simulink subsystem "FOC_Sub_CoreAlgoithm"  (R2020b)
settings: Solver=VariableStepAuto  StartTime=0.0  StopTime=10.0  RelTol=1e-3
PreLoadFcn:
  | FOC_Config;
values from neighbouring files (symbols this model uses):
  CurrentLoopMax = 1.2    [FOC_Config.m]
  fluxF = Lam_realvalue/fluxB    [FOC_Config.m]
  Id_Ki = CurrentLoopBandwidth*Rs    [FOC_Config.m]
  Id_Kp = CurrentLoopBandwidth*Ld    [FOC_Config.m]
  Iq_Ki = CurrentLoopBandwidth*Rs    [FOC_Config.m]
  Iq_Kp = CurrentLoopBandwidth*Lq    [FOC_Config.m]
  Ld = Ld_realvalue/Lb    [FOC_Config.m]
  Lq = Lq_realvalue/Lb    [FOC_Config.m]
  Omega0 = 0.4    [PLLObserver.sldd]
  PLL_KI = PLL_Bandwidth*PLL_Bandwidth    (= 0.16)    [FOC_Config.m]
  PLL_KP = 2*PLL_Bandwidth    (= 0.8)    [FOC_Config.m]
  PLL_OUTMax_W = 1.2    [FOC_Config.m]
  Rs = Rs_realvalue/Rb    [FOC_Config.m]
  tb = 1/Wb    (= 0.000636619772368)    [FOC_Config.m]
  Ts = 1/SwitchFrequency    (= 6.25e-05)    [FOC_Config.m]
  Wb = 2*pi*fn    (= 1570.79632679)    [FOC_Config.m]
undefined symbols (not defined in the file or in its folder): DiscIntNeverNeededParam, motor
libraries: mcbcontrolslib x2
settings Model: Creator=k  LastModifiedBy=wangdi

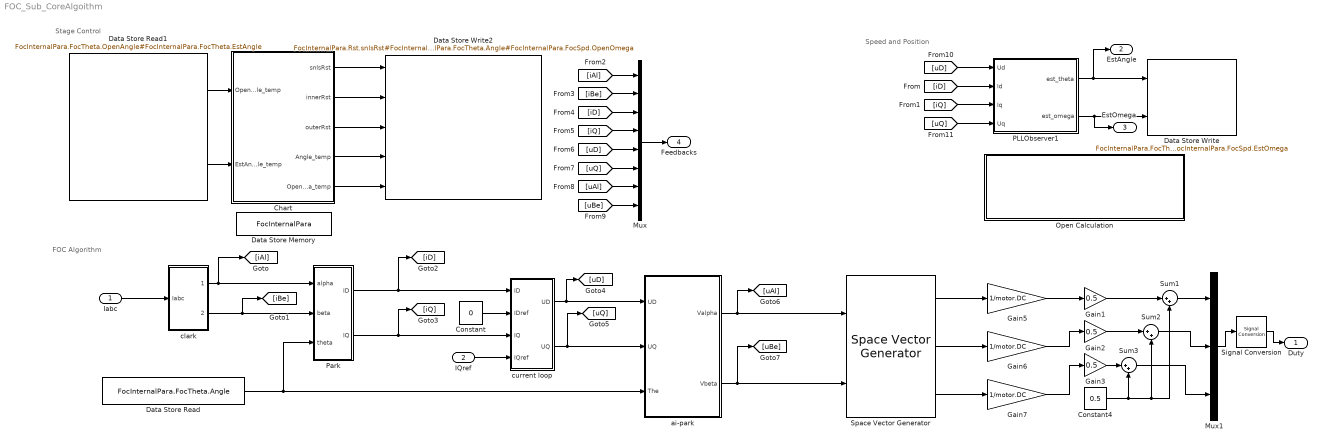
== system FOC_Sub_CoreAlgoithm ==
  note: FOC Algorithm
  note: Stage Control
  note: Speed and Position
  Iabc : Inport
  IQref : Inport  Port=2
  Chart : Stateflow chart  TreatAsAtomicUnit=on
  Constant : Constant  Value=0  OutDataTypeStr=single
  Constant4 : Constant  Value=0.5  OutDataTypeStr=single
  Data Store Memory : DataStoreMemory  DataStoreName=FocInternalPara  ReadBeforeWriteMsg=warning  WriteAfterWriteMsg=warning  WriteAfterReadMsg=warning  ShowAdditionalParam=off  OutDataTypeStr=Bus: strcutFocInternalPara
  Data Store Read : DataStoreRead  DataStoreName=FocInternalPara  DataStoreElements=FocInternalPara.FocTheta.Angle
  Data Store Read1 : DataStoreRead  DataStoreName=FocInternalPara  DataStoreElements=FocInternalPara.FocTheta.OpenAngle#FocInternalPara.FocTheta.EstAngle
  Data Store Write : DataStoreWrite  DataStoreName=FocInternalPara  DataStoreElements=FocInternalPara.FocTheta.EstAngle#FocInternalPara.FocSpd.EstOmega
  Data Store Write2 : DataStoreWrite  DataStoreName=FocInternalPara  DataStoreElements=FocInternalPara.Rst.snlsRst#FocInternalPara.Rst.innerCtrRst#FocInternalPara.Rst.outerRst#FocInternalPara.FocTheta.Angle#FocInternalPara.FocSpd.OpenOmega
  Gain1 : Gain  Gain=0.5  OutDataTypeStr=single
  Gain2 : Gain  Gain=0.5  OutDataTypeStr=single
  Gain3 : Gain  Gain=0.5  OutDataTypeStr=single
  Gain5 : Gain  Gain=1/motor.DC
  Gain6 : Gain  Gain=1/motor.DC
  Gain7 : Gain  Gain=1/motor.DC
  Mux : Mux  Inputs=8
  Mux1 : Mux  Inputs=3
  Open Calculation : Subsystem
  PLLObserver1 : Subsystem  TreatAsAtomicUnit=on
      settings: RTWFcnNameOpts=Use subsystem name  RTWFileNameOpts=Use subsystem name
  Park : Subsystem
  Signal Conversion : SignalConversion  OverrideOpt=off
  Space Vector Generator : mcbcontrolslib/Space Vector Generator
      settings: SourceProductBaseCode=MT
  Sum1 : Sum  Inputs=|++
  Sum2 : Sum  Inputs=|++
  Sum3 : Sum  Inputs=|++
  ai-park : Subsystem
  clark : Subsystem
  current loop : Subsystem
  Duty : Outport  PortDimensions=3
  EstAngle : Outport  Port=2
  EstOmega : Outport  Port=3
  Feedbacks : Outport  Port=4
  wires:
  Constant/1 -> current loop/2(IDref)
  Park/1(ID) -> [iD], current loop/1(ID)
  Iabc/1 -> clark/1(Iabc)
  Mux/1 -> Feedbacks/1
  [iAl] -> Mux/1
  [iBe] -> Mux/2
  [iD] -> Mux/3
  [iQ] -> Mux/4
  [uD] -> Mux/5
  [uQ] -> Mux/6
  [uAl] -> Mux/7
  [uBe] -> Mux/8
  [uQ] -> PLLObserver1/4(Uq)
  [uD] -> PLLObserver1/1(Ud)
  [iQ] -> PLLObserver1/3(Iq)
  [iD] -> PLLObserver1/2(Id)
  Chart/5(OpenOmega_temp) -> Data Store Write2/5
  Chart/4(Angle_temp) -> Data Store Write2/4
  Data Store Read1/2 -> Chart/2(EstAngle_temp)
  Data Store Read1/1 -> Chart/1(OpenAngle_temp)
  Chart/1(snlsRst) -> Data Store Write2/1
  Chart/2(innerRst) -> Data Store Write2/2
  Chart/3(outerRst) -> Data Store Write2/3
  Data Store Read/1 -> ai-park/3(The), Park/3(theta)
  current loop/2(UQ) -> ai-park/2(UQ), [uQ]
  current loop/1(UD) -> ai-park/1(UD), [uD]
  Park/2(IQ) -> [iQ], current loop/3(IQ)
  ai-park/2(Vbeta) -> [uBe], Space Vector Generator/2
  ai-park/1(Valpha) -> [uAl], Space Vector Generator/1
  Gain6/1 -> Gain2/1
  Gain3/1 -> Sum3/1
  Gain2/1 -> Sum2/1
  Space Vector Generator/3 -> Gain7/1
  Gain1/1 -> Sum1/1
  Gain5/1 -> Gain1/1
  Space Vector Generator/2 -> Gain6/1
  Space Vector Generator/1 -> Gain5/1
  Constant4/1 -> Sum1/2, Sum2/2, Sum3/2
  Gain7/1 -> Gain3/1
  clark/2(Ibeta) -> Park/2(beta), [iBe]
  clark/1(Ialpha) -> [iAl], Park/1(alpha)
  Sum2/1 -> Mux1/2
  Sum3/1 -> Mux1/3
  Sum1/1 -> Mux1/1
  Mux1/1 -> Signal Conversion/1
  Signal Conversion/1 -> Duty/1
  IQref/1 -> current loop/4(IQref)
  PLLObserver1/2(est_omega) -> Data Store Write/2, EstOmega/1
  PLLObserver1/1(est_theta) -> Data Store Write/1, EstAngle/1

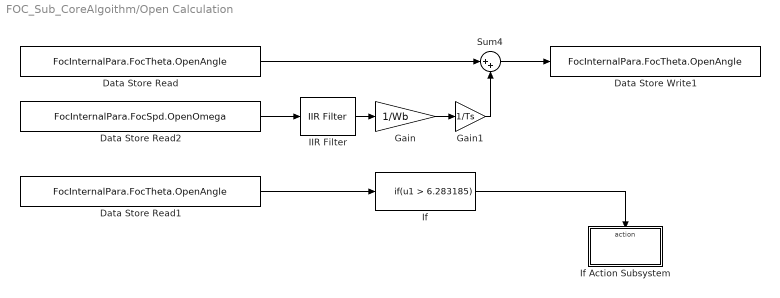
== system FOC_Sub_CoreAlgoithm/Open Calculation ==
  Data Store Read : DataStoreRead  DataStoreName=FocInternalPara  DataStoreElements=FocInternalPara.FocTheta.OpenAngle
  Data Store Read1 : DataStoreRead  DataStoreName=FocInternalPara  DataStoreElements=FocInternalPara.FocTheta.OpenAngle
  Data Store Read2 : DataStoreRead  DataStoreName=FocInternalPara  DataStoreElements=FocInternalPara.FocSpd.OpenOmega
  Data Store Write1 : DataStoreWrite  DataStoreName=FocInternalPara  DataStoreElements=FocInternalPara.FocTheta.OpenAngle
  Gain : Gain  Gain=1/Wb
  Gain1 : Gain  Gain=1/Ts
  IIR Filter : mcbcontrolslib/IIR Filter  Filter_constant=0.002
      settings: SourceProductBaseCode=MT
  If : If  IfExpression=u1 > 6.283185  ShowElse=off
  If Action Subsystem : Subsystem  TreatAsAtomicUnit=on
  Sum4 : Sum  Inputs=|++  OutDataTypeStr=single
  wires:
  Gain1/1 -> Sum4/2
  Gain/1 -> Gain1/1
  IIR Filter/1 -> Gain/1
  Data Store Read2/1 -> IIR Filter/1
  Sum4/1 -> Data Store Write1/1
  Data Store Read/1 -> Sum4/1
  Data Store Read1/1 -> If/1
  If/1 -> If Action Subsystem/Action

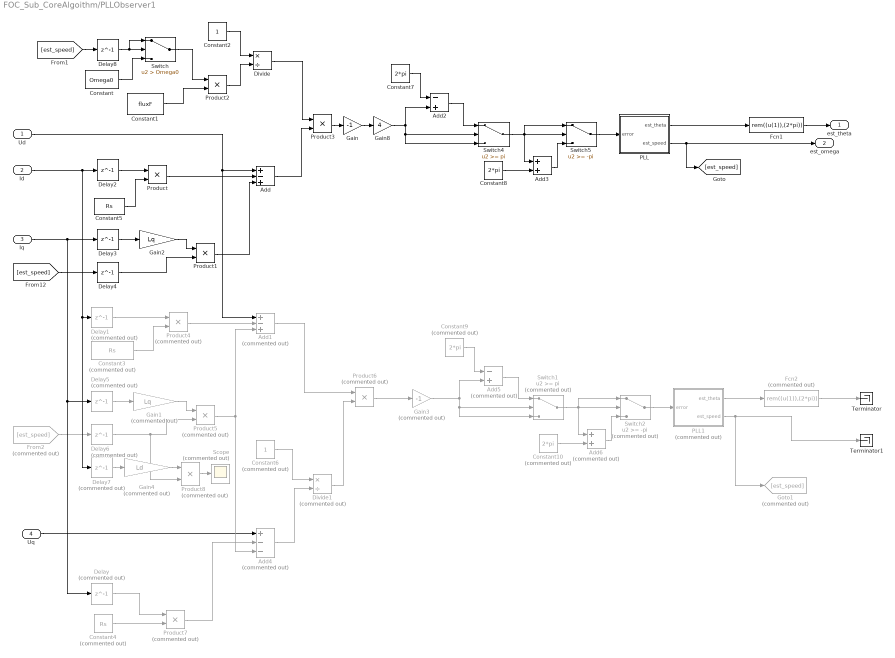
== system FOC_Sub_CoreAlgoithm/PLLObserver1 ==
  Ud : Inport
  Id : Inport  Port=2
  Iq : Inport  Port=3
  Uq : Inport  Port=4
  Add : Sum  Inputs=+-+
  Add1 : Sum  Commented=on  Inputs=+-+
  Add2 : Sum  Inputs=-+
  Add3 : Sum
  Add4 : Sum  Commented=on  Inputs=+--
  Add5 : Sum  Commented=on  Inputs=-+
  Add6 : Sum  Commented=on
  Constant : Constant  Value=Omega0  OutDataTypeStr=single
  Constant1 : Constant  Value=fluxF  OutDataTypeStr=single
  Constant10 : Constant  Commented=on  Value=2*pi
  Constant2 : Constant  OutDataTypeStr=single
  Constant3 : Constant  Commented=on  Value=Rs  OutDataTypeStr=single
  Constant4 : Constant  Commented=on  Value=Rs  OutDataTypeStr=single
  Constant5 : Constant  Value=Rs  OutDataTypeStr=single
  Constant6 : Constant  Commented=on  OutDataTypeStr=single
  Constant7 : Constant  Value=2*pi  OutDataTypeStr=single
  Constant8 : Constant  Value=2*pi  OutDataTypeStr=single
  Constant9 : Constant  Commented=on  Value=2*pi  OutDataTypeStr=single
  Delay{,1,5..7} (5 alike) : Delay  Commented=on  DelayLength=1
  Delay{2..4,8} (4 alike) : Delay  DelayLength=1
  Divide : Product  Inputs=*/
  Divide1 : Product  Commented=on  Inputs=*/
  Fcn1 : Fcn  Expr=rem((u(1)),(2*pi))
  Fcn2 : Fcn  Commented=on  Expr=rem((u(1)),(2*pi))
  From2 : From  Commented=on  GotoTag=est_speed
  Gain : Gain  Gain=-1
  Gain1 : Gain  Commented=on  Gain=Lq
  Gain2 : Gain  Gain=Lq
  Gain3 : Gain  Commented=on  Gain=-1
  Gain4 : Gain  Commented=on  Gain=Ld
  Gain8 : Gain  Gain=4
  Goto1 : Goto  Commented=on  GotoTag=est_speed
  PLL : Subsystem  TreatAsAtomicUnit=on
  PLL1 : Subsystem  Commented=on
  Product{,1..3} (4 alike) : Product
  Product{4..8} (5 alike) : Product  Commented=on
  Scope : Scope  Commented=on
  Switch : Switch  Criteria=u2 > Threshold  Threshold=Omega0
  Switch1 : Switch  Commented=on  Threshold=pi
  Switch2 : Switch  Commented=on  Threshold=-pi
  Switch4 : Switch  Threshold=pi
  Switch5 : Switch  Threshold=-pi
  Terminator : Terminator
  Terminator1 : Terminator
  est_theta : Outport
  est_omega : Outport  Port=2
  wires:
  [est_speed] -> Delay8/1
  PLL/1(est_theta) -> Fcn1/1
  Gain8/1 -> Add2/2, Switch4/2, Switch4/3
  Add/1 -> Product3/2
  Product1/1 -> Add/3
  Product/1 -> Add/2
  Product8/1 -> Scope/1
  Gain4/1 -> Product8/1
  From2/1 -> Delay6/1
  Delay7/1 -> Gain4/1
  Fcn1/1 -> est_theta/1
  PLL1/2(est_speed) -> Goto1/1, Terminator1/1
  Fcn2/1 -> Terminator/1
  PLL1/1(est_theta) -> Fcn2/1
  Add6/1 -> Switch2/3
  Gain3/1 -> Add5/2, Switch1/2, Switch1/3
  Add5/1 -> Switch1/1
  Switch2/1 -> PLL1/1(error)
  Constant10/1 -> Add6/2
  Constant9/1 -> Add5/1
  Switch1/1 -> Switch2/2, Add6/1, Switch2/1
  Product6/1 -> Gain3/1
  Divide1/1 -> Product6/2
  Add4/1 -> Divide1/2
  Constant6/1 -> Divide1/1
  Product7/1 -> Add4/2
  Constant4/1 -> Product7/2
  Delay/1 -> Product7/1
  Uq/1 -> Add4/1
  Add1/1 -> Product6/1
  Product5/1 -> Add1/3, Add4/3
  Iq/1 -> Delay3/1, Delay5/1, Delay/1
  Delay5/1 -> Gain1/1
  Gain1/1 -> Product5/1
  Delay6/1 -> Product5/2, Product8/2
  Ud/1 -> Add/1, Add1/1
  Delay1/1 -> Product4/1
  Product4/1 -> Add1/2
  Constant3/1 -> Product4/2
  Gain/1 -> Gain8/1
  Product3/1 -> Gain/1
  Switch5/1 -> PLL/1(error)
  Add2/1 -> Switch4/1
  Constant7/1 -> Add2/1
  Constant8/1 -> Add3/2
  Add3/1 -> Switch5/3
  PLL/2(est_speed) -> [est_speed], est_omega/1
  Switch4/1 -> Switch5/2, Add3/1, Switch5/1
  Divide/1 -> Product3/1
  Product2/1 -> Divide/2
  Constant2/1 -> Divide/1
  Constant1/1 -> Product2/2
  Switch/1 -> Product2/1
  Constant/1 -> Switch/3
  Delay8/1 -> Switch/2, Switch/1
  Id/1 -> Delay2/1, Delay1/1, Delay7/1
  Delay2/1 -> Product/1
  Delay3/1 -> Gain2/1
  Gain2/1 -> Product1/1
  Delay4/1 -> Product1/2
  [est_speed] -> Delay4/1
  Constant5/1 -> Product/2

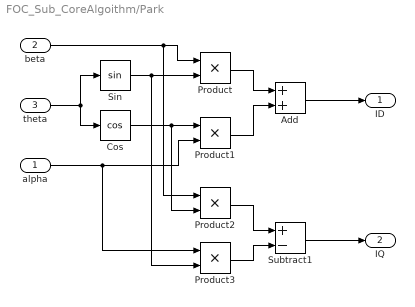
== system FOC_Sub_CoreAlgoithm/Park ==
  alpha : Inport
  beta : Inport  Port=2
  theta : Inport  Port=3
  Add : Sum  OutDataTypeStr=single
  Cos : Trigonometry  Operator=cos
  Product{,1..3} (4 alike) : Product
  Sin : Trigonometry
  Subtract1 : Sum  Inputs=+-  OutDataTypeStr=single
  ID : Outport
  IQ : Outport  Port=2
  wires:
  Product2/1 -> Subtract1/1
  beta/1 -> Product2/1, Product/1
  theta/1 -> Cos/1, Sin/1
  Sin/1 -> Product3/2, Product/2
  alpha/1 -> Product3/1, Product1/2
  Cos/1 -> Product1/1, Product2/2
  Subtract1/1 -> IQ/1
  Product1/1 -> Add/2
  Product3/1 -> Subtract1/2
  Product/1 -> Add/1
  Add/1 -> ID/1

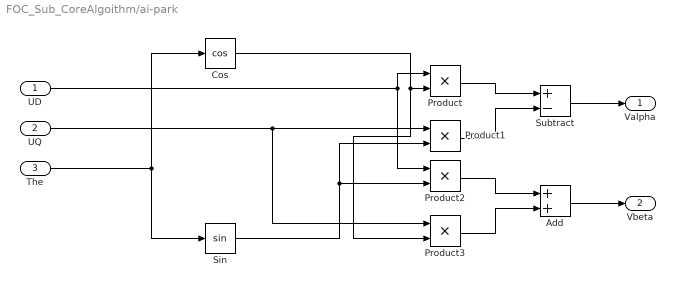
== system FOC_Sub_CoreAlgoithm/ai-park ==
  UD : Inport
  UQ : Inport  Port=2
  The : Inport  Port=3
  Add : Sum
  Cos : Trigonometry  Operator=cos
  Product{,1..3} (4 alike) : Product
  Sin : Trigonometry
  Subtract : Sum  Inputs=+-
  Valpha : Outport
  Vbeta : Outport  Port=2
  wires:
  Add/1 -> Vbeta/1
  Subtract/1 -> Valpha/1
  UD/1 -> Product2/1, Product/1
  The/1 -> Cos/1, Sin/1
  Product2/1 -> Add/1
  Product/1 -> Subtract/1
  Sin/1 -> Product1/2, Product2/2
  Cos/1 -> Product/2, Product3/2
  Product3/1 -> Add/2
  Product1/1 -> Subtract/2
  UQ/1 -> Product1/1, Product3/1

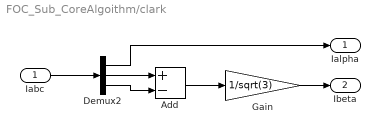
== system FOC_Sub_CoreAlgoithm/clark ==
  Iabc : Inport  OutDataTypeStr=single
  Add : Sum  Inputs=+-
  Demux2 : Demux  Outputs=3
  Gain : Gain  Gain=1/sqrt(3)
  Ialpha : Outport
  Ibeta : Outport  Port=2
  wires:
  Demux2/3 -> Add/2
  Demux2/1 -> Ialpha/1
  Demux2/2 -> Add/1
  Iabc/1 -> Demux2/1
  Add/1 -> Gain/1
  Gain/1 -> Ibeta/1

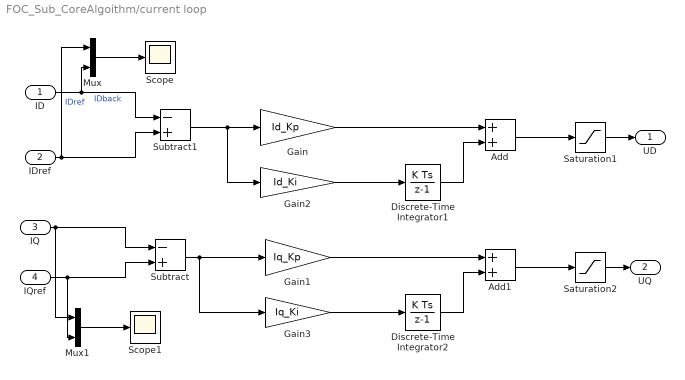
== system FOC_Sub_CoreAlgoithm/current loop ==
  ID : Inport  OutDataTypeStr=single
  IDref : Inport  Port=2  OutDataTypeStr=single
  IQ : Inport  Port=3  OutDataTypeStr=single
  IQref : Inport  Port=4  OutDataTypeStr=single
  Add : Sum
  Add1 : Sum
  Discrete-Time Integrator1 : DiscreteIntegrator  gainval=1/tb  SampleTime=-1  LimitOutput=on  UpperSaturationLimit=CurrentLoopMax  LowerSaturationLimit=-CurrentLoopMax  ICPrevOutput=DiscIntNeverNeededParam  ICPrevScaledInput=DiscIntNeverNeededParam
  Discrete-Time Integrator2 : DiscreteIntegrator  gainval=1/tb  SampleTime=-1  LimitOutput=on  UpperSaturationLimit=CurrentLoopMax  LowerSaturationLimit=-CurrentLoopMax  ICPrevOutput=DiscIntNeverNeededParam  ICPrevScaledInput=DiscIntNeverNeededParam
  Gain : Gain  Gain=Id_Kp
  Gain1 : Gain  Gain=Iq_Kp
  Gain2 : Gain  Gain=Id_Ki
  Gain3 : Gain  Gain=Iq_Ki
  Mux : Mux  Inputs=2
  Mux1 : Mux  Inputs=2
  Saturation1 : Saturate  UpperLimit=CurrentLoopMax  LowerLimit=-CurrentLoopMax
  Saturation2 : Saturate  UpperLimit=CurrentLoopMax  LowerLimit=-CurrentLoopMax
  Scope : Scope
  Scope1 : Scope
  Subtract : Sum  Inputs=-+
  Subtract1 : Sum  Inputs=-+
  UD : Outport
  UQ : Outport  Port=2
  wires:
  Saturation1/1 -> UD/1
  Subtract1/1 -> Gain/1, Gain2/1
  Saturation2/1 -> UQ/1
  Subtract/1 -> Gain3/1, Gain1/1
  Discrete-Time Integrator1/1 -> Add/2
  Discrete-Time Integrator2/1 -> Add1/2
  IQref/1 -> Mux1/2, Subtract/2
  IDref/1 -> Mux/1, Subtract1/2  "IDref"
  ID/1 -> Mux/2, Subtract1/1  "IDback"
  Mux/1 -> Scope/1
  IQ/1 -> Mux1/1, Subtract/1
  Mux1/1 -> Scope1/1
  Add/1 -> Saturation1/1
  Add1/1 -> Saturation2/1
  Gain1/1 -> Add1/1
  Gain3/1 -> Discrete-Time Integrator2/1
  Gain/1 -> Add/1
  Gain2/1 -> Discrete-Time Integrator1/1

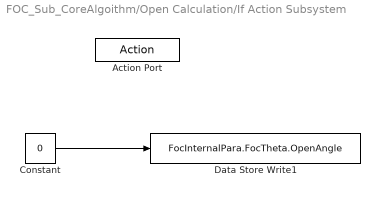
== system FOC_Sub_CoreAlgoithm/Open Calculation/If Action Subsystem ==
  Action Port : ActionPort
  Constant : Constant  Value=0  OutDataTypeStr=single
  Data Store Write1 : DataStoreWrite  DataStoreName=FocInternalPara  DataStoreElements=FocInternalPara.FocTheta.OpenAngle
  wires:
  Constant/1 -> Data Store Write1/1

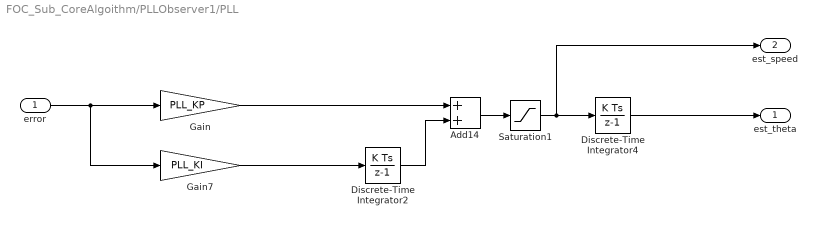
== system FOC_Sub_CoreAlgoithm/PLLObserver1/PLL ==
  error : Inport
  Add14 : Sum
  Discrete-Time Integrator2 : DiscreteIntegrator  gainval=1  SampleTime=-1  LimitOutput=on  UpperSaturationLimit=PLL_OUTMax_W  LowerSaturationLimit=-PLL_OUTMax_W  ICPrevOutput=DiscIntNeverNeededParam  ICPrevScaledInput=DiscIntNeverNeededParam
  Discrete-Time Integrator4 : DiscreteIntegrator  gainval=1.0/tb  SampleTime=-1  UpperSaturationLimit=PLL_OUTMax_W  LowerSaturationLimit=-PLL_OUTMax_W  ICPrevOutput=DiscIntNeverNeededParam  ICPrevScaledInput=DiscIntNeverNeededParam
  Gain : Gain  Gain=PLL_KP
  Gain7 : Gain  Gain=PLL_KI
  Saturation1 : Saturate  UpperLimit=PLL_OUTMax_W  LowerLimit=-PLL_OUTMax_W
  est_theta : Outport
  est_speed : Outport  Port=2
  wires:
  Discrete-Time Integrator4/1 -> est_theta/1
  Gain7/1 -> Discrete-Time Integrator2/1
  Gain/1 -> Add14/1
  Discrete-Time Integrator2/1 -> Add14/2
  error/1 -> Gain/1, Gain7/1
  Saturation1/1 -> Discrete-Time Integrator4/1, est_speed/1
  Add14/1 -> Saturation1/1

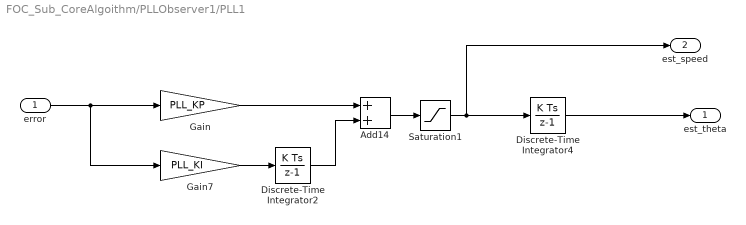
== system FOC_Sub_CoreAlgoithm/PLLObserver1/PLL1 ==
  error : Inport
  Add14 : Sum
  Discrete-Time Integrator2 : DiscreteIntegrator  gainval=1.0/tb  SampleTime=-1  LimitOutput=on  UpperSaturationLimit=PLL_OUTMax_W  LowerSaturationLimit=-PLL_OUTMax_W  ICPrevOutput=DiscIntNeverNeededParam  ICPrevScaledInput=DiscIntNeverNeededParam
  Discrete-Time Integrator4 : DiscreteIntegrator  gainval=1.0/tb  SampleTime=-1  UpperSaturationLimit=PLL_OUTMax_W  LowerSaturationLimit=-PLL_OUTMax_W  ICPrevOutput=DiscIntNeverNeededParam  ICPrevScaledInput=DiscIntNeverNeededParam
  Gain : Gain  Gain=PLL_KP
  Gain7 : Gain  Gain=PLL_KI
  Saturation1 : Saturate  UpperLimit=PLL_OUTMax_W  LowerLimit=-PLL_OUTMax_W
  est_theta : Outport
  est_speed : Outport  Port=2
  wires:
  Gain/1 -> Add14/1
  Discrete-Time Integrator2/1 -> Add14/2
  error/1 -> Gain/1, Gain7/1
  Saturation1/1 -> Discrete-Time Integrator4/1, est_speed/1
  Add14/1 -> Saturation1/1
  Discrete-Time Integrator4/1 -> est_theta/1
  Gain7/1 -> Discrete-Time Integrator2/1

== stateflow chart FOC_Sub_CoreAlgoithm/Chart ==
  state OpenStage
    outerRst = 1;
    snlsRst = 1;
    innerRst = 0;
    Angle_temp = OpenAngle_temp;
    OpenOmega_temp = 94;
  state RunStage
    outerRst = 0;
    snlsRst = 0;
    innerRst = 0;
    Angle_temp = EstAngle_temp;
    OpenOmega_temp = 0;
  state AlignStage
    outerRst = 1;
    snlsRst = 1;
    innerRst = 1;
    Angle_temp = 0;
    OpenOmega_temp = 0;
  state TrackStage
    outerRst = 1;
    snlsRst = 0;
    innerRst = 0;
    Angle_temp = OpenAngle_temp;
    OpenOmega_temp = 94;
  (default) -> AlignStage
  OpenStage -> TrackStage : after(8000, tick)
  AlignStage -> OpenStage : after(8000, tick)
  TrackStage -> RunStage : after(20000, tick)
  data: snlsRst output single; innerRst output single; outerRst output single; OpenAngle_temp input single; EstAngle_temp input single; Angle_temp output single; OpenOmega_temp output single
